simulink model "Camera_modifiedMaass"  (Simulink 7.3)
settings: Solver=FixedStepDiscrete  StartTime=0.0  StopTime=inf  FixedStep=0.1  RelTol=1e-3
libraries: simulink x11, xpclib x2
settings Model: Creator=atlabor  LastModifiedBy=RobotScout
settings MATStruct: SampleTime=0.1  Offset=0  Priority=[10000000.0]
settings DataIOCC: MaxDataPoints=5000
settings HardwareCC: ProdHWDeviceType=Generic->Unspecified (assume 32-bit Generic)

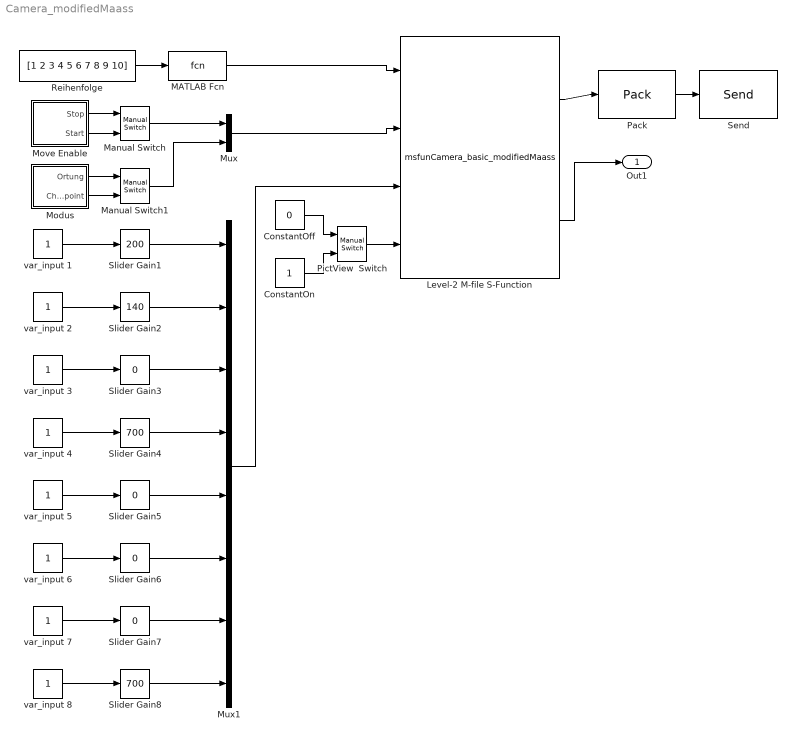
== system Camera_modifiedMaass ==
  ConstantOff : Constant  Value=0  OutDataType=fixdt(1, 16)  OutScaling=2^0
  ConstantOn : Constant  OutDataType=fixdt(1, 16)  OutScaling=2^0
  Level-2 M-file S-Function : M-S-Function  FunctionName=msfunCamera_basic_modifiedMaass
  MATLAB Fcn : MATLABFcn  MATLABFcn=fcn  OutputDimensions=10
  Manual Switch : simulink/Signal Routing/Manual Switch  SystemSampleTime=-1  sw=1  action=0  varsize=off
  Manual Switch1 : simulink/Signal Routing/Manual Switch  SystemSampleTime=-1  sw=1  action=0  varsize=off
  Modus : Subsystem
  Move Enable : Subsystem
  Mux : Mux  Inputs=2
  Mux1 : Mux  Inputs=8
  Pack : xpclib/UDP/Pack  datatypes={'double'}  byteAlign=1
  PictView  Switch : simulink/Signal Routing/Manual Switch  SystemSampleTime=-1  sw=0  action=0  varsize=off
  Reihenfolge : Constant  Value=[1 2 3 4 5 6 7 8 9 10]  VectorParams1D=off  OutDataType=fixdt(1, 16)  OutScaling=2^0
  Send : xpclib/UDP/Send  ipAddress=255.255.255.255  ipPort=25000  localPort=-1  sampletime=-1
  Slider Gain1 : simulink/Math Operations/Slider Gain  SystemSampleTime=-1  low=0  gain=200  high=500
  Slider Gain2 : simulink/Math Operations/Slider Gain  SystemSampleTime=-1  low=-200  gain=140  high=200
  Slider Gain{3,5..7} (4 alike) : simulink/Math Operations/Slider Gain  SystemSampleTime=-1  low=0  gain=0  high=800
  Slider Gain4 : simulink/Math Operations/Slider Gain  SystemSampleTime=-1  low=500  gain=700  high=1000
  Slider Gain8 : simulink/Math Operations/Slider Gain  SystemSampleTime=-1  low=500  gain=700  high=900
  var_input {1..8} (8 alike) : Constant  OutDataType=fixdt(1, 16)  OutScaling=2^0
  Out1 : Outport  OutDataType=fixdt(1, 16)  OutScaling=2^0
  wires:
  Level-2 M-file S-Function/1 -> Pack/1
  Pack/1 -> Send/1
  Move Enable/1(Stop) -> Manual Switch/1
  Move Enable/2(Start) -> Manual Switch/2
  Modus/1(Ortung) -> Manual Switch1/1
  Modus/2(Checkpoint) -> Manual Switch1/2
  Manual Switch/1 -> Mux/1
  Manual Switch1/1 -> Mux/2
  var_input 1/1 -> Slider Gain1/1
  Slider Gain1/1 -> Mux1/1
  var_input 2/1 -> Slider Gain2/1
  var_input 3/1 -> Slider Gain3/1
  var_input 4/1 -> Slider Gain4/1
  var_input 5/1 -> Slider Gain5/1
  var_input 6/1 -> Slider Gain6/1
  var_input 7/1 -> Slider Gain7/1
  var_input 8/1 -> Slider Gain8/1
  Slider Gain8/1 -> Mux1/8
  Slider Gain2/1 -> Mux1/2
  Slider Gain3/1 -> Mux1/3
  Slider Gain4/1 -> Mux1/4
  Slider Gain5/1 -> Mux1/5
  Slider Gain6/1 -> Mux1/6
  Slider Gain7/1 -> Mux1/7
  Mux/1 -> Level-2 M-file S-Function/2
  Mux1/1 -> Level-2 M-file S-Function/3
  Level-2 M-file S-Function/2 -> Out1/1
  MATLAB Fcn/1 -> Level-2 M-file S-Function/1
  Reihenfolge/1 -> MATLAB Fcn/1
  PictView  Switch/1 -> Level-2 M-file S-Function/4
  ConstantOn/1 -> PictView  Switch/2
  ConstantOff/1 -> PictView  Switch/1

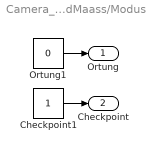
== system Camera_modifiedMaass/Modus ==
  Checkpoint1 : Constant  OutDataType=fixdt(1, 16)  OutScaling=2^0
  Ortung1 : Constant  Value=0  OutDataType=fixdt(1, 16)  OutScaling=2^0
  Ortung : Outport
  Checkpoint : Outport  Port=2
  wires:
  Ortung1/1 -> Ortung/1
  Checkpoint1/1 -> Checkpoint/1

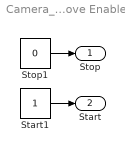
== system Camera_modifiedMaass/Move Enable ==
  Start1 : Constant  OutDataType=fixdt(1, 16)  OutScaling=2^0
  Stop1 : Constant  Value=0  OutDataType=fixdt(1, 16)  OutScaling=2^0
  Stop : Outport
  Start : Outport  Port=2
  wires:
  Stop1/1 -> Stop/1
  Start1/1 -> Start/1
